simulink model "cartesianLinearYA"  (R2023a)
settings: Solver=ode4  StartTime=0.0  StopTime=10.0  FixedStep=dt  RelTol=1e-3
settings Model: Creator=ndelurgio  LastModifiedBy=ndelurgio

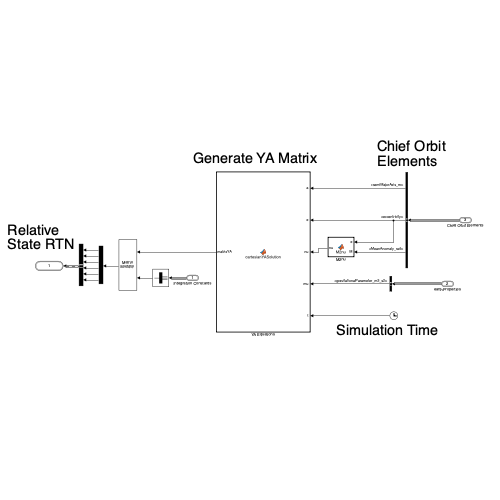
[thumbnail: Simulink's stored preview of the top-level diagram]
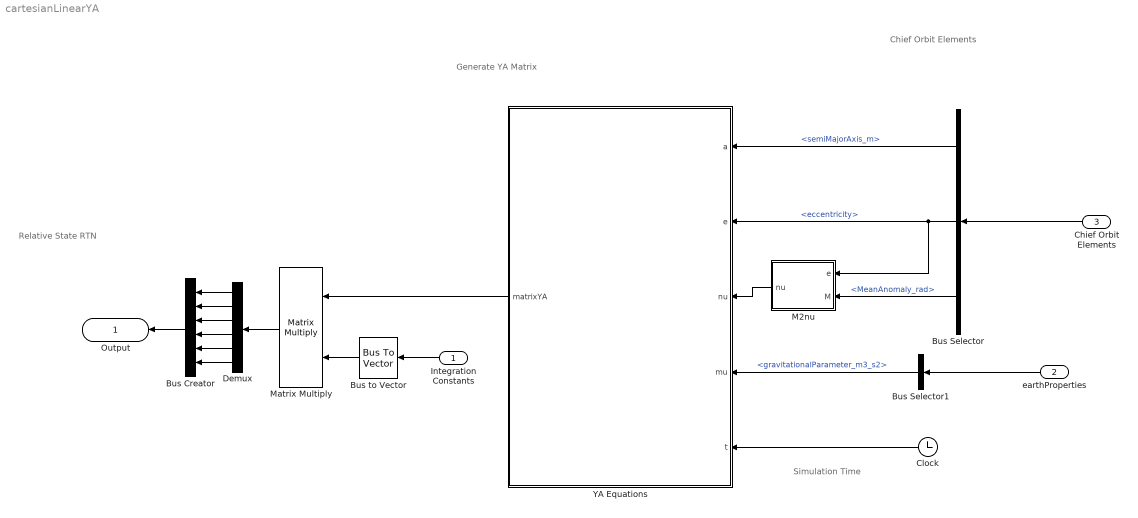
== system cartesianLinearYA ==
  note: Simulation Time
  note: Generate YA Matrix
  note: Relative State RTN
  note: Chief Orbit Elements
  Integration Constants : Inport  OutDataTypeStr=Bus: integrationConstants_YA
  earthProperties : Inport  Port=2  OutDataTypeStr=Bus: earthProperties
  Chief Orbit Elements : Inport  Port=3  OutDataTypeStr=Bus: meanOrbitElements
  Bus Creator : BusCreator  Inputs=6  OutDataTypeStr=Bus: relativeCartesianState  NonVirtualBus=on
      settings: InheritFromInputs=off
  Bus Selector : BusSelector  OutputSignals=semiMajorAxis_m,eccentricity,MeanAnomaly_rad
  Bus Selector1 : BusSelector  OutputSignals=gravitationalParameter_m3_s2
  Bus to Vector : BusToVector
  Clock : Clock
  Demux : Demux  Outputs=6
  M2nu : MATLAB Function  TreatAsAtomicUnit=on
  Matrix Multiply : Product  Multiplication=Matrix(*)
  YA Equations : MATLAB Function  TreatAsAtomicUnit=on
  Output : Outport  OutDataTypeStr=Bus: relativeCartesianState
  wires:
  Integration Constants/1 -> Bus to Vector/1
  Chief Orbit Elements/1 -> Bus Selector/1
  Bus Selector/1 -> YA Equations/1(a)  "<semiMajorAxis_m>"
  earthProperties/1 -> Bus Selector1/1
  Bus Selector1/1 -> YA Equations/4(mu)  "<gravitationalParameter_m3_s2>"
  Clock/1 -> YA Equations/5(t)
  YA Equations/1(matrixYA) -> Matrix Multiply/1
  Demux/1 -> Bus Creator/1
  Demux/2 -> Bus Creator/2
  Demux/3 -> Bus Creator/3
  Demux/4 -> Bus Creator/4
  Demux/5 -> Bus Creator/5
  Demux/6 -> Bus Creator/6
  Bus Creator/1 -> Output/1
  Matrix Multiply/1 -> Demux/1
  Bus to Vector/1 -> Matrix Multiply/2
  Bus Selector/2 -> YA Equations/2(e), M2nu/1(e)  "<eccentricity>"
  M2nu/1(nu) -> YA Equations/3(nu)
  Bus Selector/3 -> M2nu/2(M)  "<MeanAnomaly_rad>"

== matlab function cartesianLinearYA/M2nu ==
  data: e input; M input; nu output
function nu = M2nu(e,M)
nu = M2nu(M,e);
end

== matlab function cartesianLinearYA/YA Equations ==
  data: matrixYA output; a input; e input; nu input; mu input; t input
function matrixYA = cartesianYASolution(a, e, nu, mu, t)

matrixYA = cartesianYASolution(a, e, nu, t, mu);

end
